simulink model "problem_3"  (R2018a)
settings: Solver=VariableStepAuto  StartTime=0.0  StopTime=10  MaxStep=1e-3  RelTol=1e-3
values from neighbouring files (symbols this model uses):
  a0 = 68 * pi/180    (= 1.18682389136)    [grid_search_minimization.m]    (also in minimization.m = a0Vec(aIdx); problem_1_script.m; problem_3_script.m; smm_params.m)
  dx0 = 1.123    [distance_x.m]    (also in grid_search_minimization.m = sqrt(2/m*(Esys-m*g*y0)); minimization.m = sqrt(2/m*(Esys-m*g*y0)); problem_1_script.m = 5; problem_3_script.m = sqrt(2/m*(Esys-m*g*y0)))
  dy0 = 0    [distance_x.m]    (also in grid_search_minimization.m; minimization.m; problem_1_script.m; problem_3_script.m)
  g = 9.81    [distance_x.m]    (also in grid_search_minimization.m; minimization.m; problem_1_script.m; problem_3_script.m)
  l0 = 0.9937    [distance_x.m]    (also in grid_search_minimization.m = 1; minimization.m = 1; problem_1_script.m = 1; problem_3_script.m = 1)
  m = 80    [distance_x.m]    (also in grid_search_minimization.m; minimization.m; problem_1_script.m; problem_3_script.m)
  x0 = 0    [distance_x.m]    (also in grid_search_minimization.m; minimization.m; problem_1_script.m; problem_3_script.m)
  y0 = l0    (= 0.9937)    [distance_x.m]    (also in grid_search_minimization.m = y0Vec(yIdx); minimization.m = y0Vec(yIdx); problem_1_script.m = 1; problem_3_script.m = y0Vec3(yIdx))
libraries: simulink_extras x1
settings Model: Creator=hgeyer  LastModifiedBy=oliver

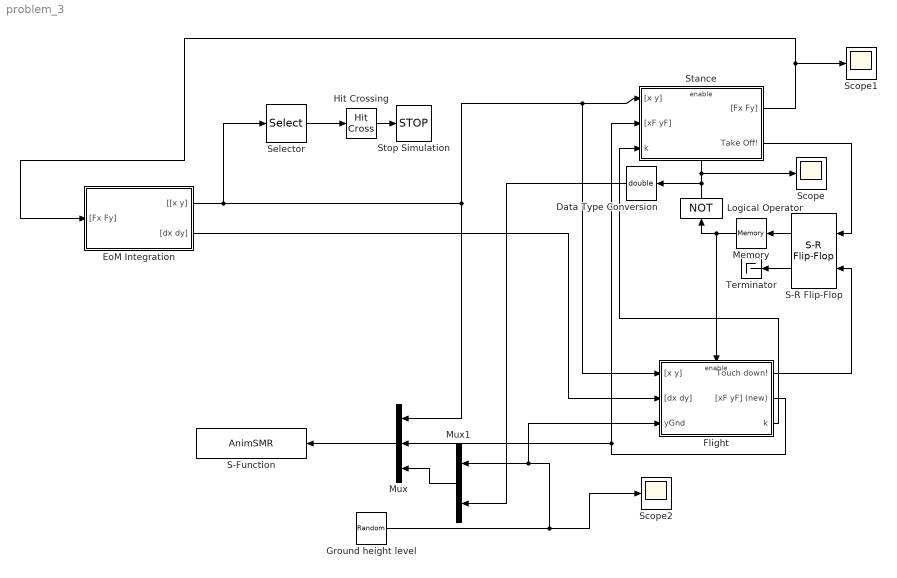
== system problem_3 ==
  " Stance" : Subsystem
  Data Type Conversion : DataTypeConversion  OutDataTypeStr=double
  EoM Integration : Subsystem
  Flight : Subsystem
  Ground height level : UniformRandomNumber  Minimum=-.02  Maximum=.02  SampleTime=0.3
  Hit Crossing : HitCross  HitCrossingDirection=falling
  Logical Operator : Logic  Operator=NOT  AllPortsSameDT=off  OutDataTypeStr=boolean
  Memory : Memory  InitialCondition=1
  Mux : Mux  Inputs=3
  Mux1 : Mux  Inputs=2
  S-Function : S-Function  FunctionName=AnimSMR  Parameters=0.01  SFunctionDeploymentMode=off  EnableBusSupport=off
  S-R Flip-Flop : simulink_extras/Flip Flops/S-R Flip-Flop  initial_condition=1
  Scope : Scope
  Scope1 : Scope
  Scope2 : Scope
  Selector : Selector  InputPortWidth=2  IndexOptions=Index vector (dialog)  Indices=[2]  OutputSizes=1
  Stop Simulation : Stop
  Terminator : Terminator
  wires:
  EoM Integration/1("[[x y]") -> Selector/1, Flight/1("[x y]"), " Stance"/1("[x y]"), Mux/1
  EoM Integration/2("[dx dy]") -> Flight/2("[dx dy]")
  " Stance"/2(Take Off!) -> S-R Flip-Flop/1
  S-R Flip-Flop/1 -> Memory/1
  Logical Operator/1 -> Data Type Conversion/1, " Stance"/Enable, Scope/1
  Memory/1 -> Logical Operator/1, Flight/Enable
  S-R Flip-Flop/2 -> Terminator/1
  Flight/1(Touch down!) -> S-R Flip-Flop/2
  " Stance"/1("[Fx Fy]") -> EoM Integration/1("[Fx Fy]"), Scope1/1
  Flight/2("[xF yF] (new)") -> " Stance"/2("[xF yF]"), Mux/2
  Mux/1 -> S-Function/1
  Mux1/1 -> Mux/3
  Data Type Conversion/1 -> Mux1/2
  Ground height level/1 -> Flight/3(yGnd), Mux1/1, Scope2/1
  Hit Crossing/1 -> Stop Simulation/1
  Selector/1 -> Hit Crossing/1
  Flight/3(k) -> " Stance"/3(k)

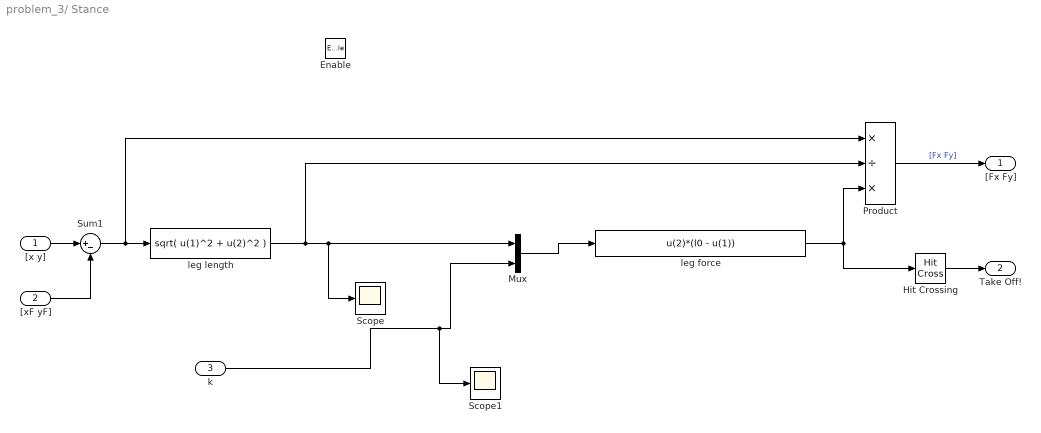
== system problem_3/ Stance ==
  "[x y]" : Inport
  "[xF yF]" : Inport  Port=2
  k : Inport  Port=3
  Enable : EnablePort
  Hit Crossing : HitCross  HitCrossingDirection=falling
  Mux : Mux  Inputs=2
  Product : Product  Inputs=*/*
  Scope : Scope
  Scope1 : Scope
  Sum1 : Sum  Inputs=|+-
  leg force : Fcn  Expr=u(2)*(l0 - u(1))
  leg length : Fcn  Expr=sqrt( u(1)^2 + u(2)^2 )
  "[Fx Fy]" : Outport  OutputWhenDisabled=reset  InitialOutput=[0,0]
  Take Off! : Outport  Port=2  OutputWhenDisabled=reset  InitialOutput=0
  wires:
  Product/1 -> "[Fx Fy]"/1  "[Fx Fy]"
  leg length/1 -> Scope/1, Mux/1, Product/2
  Hit Crossing/1 -> Take Off!/1
  "[x y]"/1 -> Sum1/1
  "[xF yF]"/1 -> Sum1/2
  Sum1/1 -> Product/1, leg length/1
  leg force/1 -> Hit Crossing/1, Product/3
  k/1 -> Scope1/1, Mux/2
  Mux/1 -> leg force/1

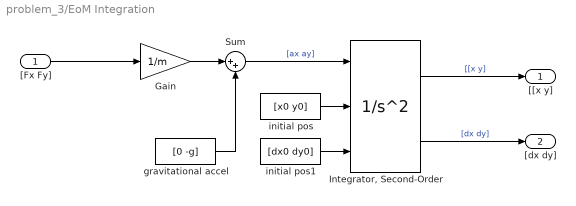
== system problem_3/EoM Integration ==
  "[Fx Fy]" : Inport
  Gain : Gain  Gain=1/m
  "Integrator, Second-Order" : SecondOrderIntegrator  ICSourceX=external  ICSourceDXDT=external
  Sum : Sum  Inputs=|++
  gravitational accel : Constant  Value=[0 -g]
  initial pos : Constant  Value=[x0 y0]
  initial pos1 : Constant  Value=[dx0 dy0]
  "[[x y]" : Outport
  "[dx dy]" : Outport  Port=2
  wires:
  "[Fx Fy]"/1 -> Gain/1
  initial pos1/1 -> "Integrator, Second-Order"/3
  "Integrator, Second-Order"/2 -> "[dx dy]"/1  "[dx dy]"
  Gain/1 -> Sum/1
  initial pos/1 -> "Integrator, Second-Order"/2
  "Integrator, Second-Order"/1 -> "[[x y]"/1  "[[x y]"
  Sum/1 -> "Integrator, Second-Order"/1  "[ax ay]"
  gravitational accel/1 -> Sum/2

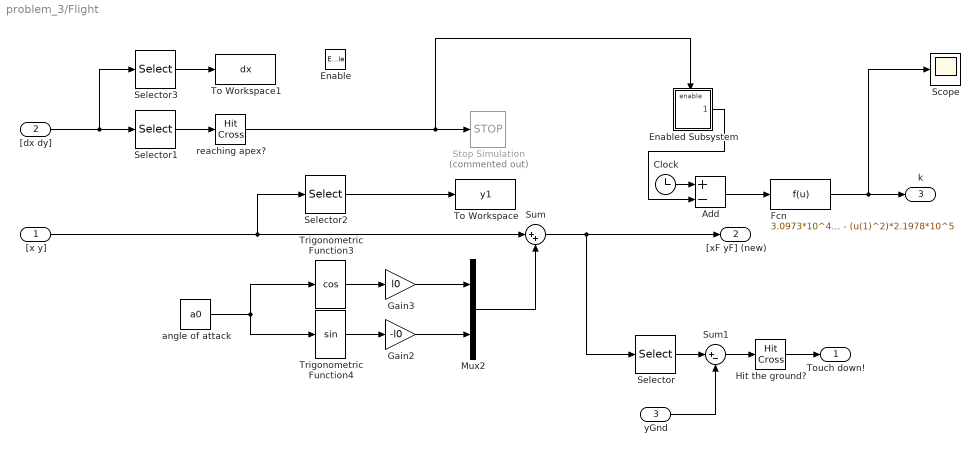
== system problem_3/Flight ==
  "[x y]" : Inport
  "[dx dy]" : Inport  Port=2
  yGnd : Inport  Port=3
  Enable : EnablePort
  Add : Sum  Inputs=+-
  Clock : Clock
  Enabled Subsystem : Subsystem  TreatAsAtomicUnit=on
  Fcn : Fcn  Expr=3.0973*10^4 - (u(1)^2)*2.1978*10^5
  Gain2 : Gain  Gain=-l0
  Gain3 : Gain  Gain=l0
  Hit the ground? : HitCross  HitCrossingDirection=falling
  Mux2 : Mux  Inputs=2
  Scope : Scope
  Selector : Selector  InputPortWidth=2  IndexOptions=Index vector (dialog)  Indices=2  OutputSizes=1
  Selector1 : Selector  InputPortWidth=2  IndexOptions=Index vector (dialog)  Indices=2  OutputSizes=1
  Selector2 : Selector  InputPortWidth=2  IndexOptions=Index vector (dialog)  Indices=2  OutputSizes=1
  Selector3 : Selector  InputPortWidth=2  IndexOptions=Index vector (dialog)  Indices=1  OutputSizes=1
  Stop Simulation : Stop  Commented=on
  Sum : Sum  Inputs=|++
  Sum1 : Sum  Inputs=|+-
  To Workspace : ToWorkspace  VariableName=y1  SampleTime=-1
      settings: MaxDataPoints=1
  To Workspace1 : ToWorkspace  VariableName=dx  SampleTime=-1
  Trigonometric Function3 : Trigonometry  Operator=cos
  Trigonometric Function4 : Trigonometry
  angle of attack : Constant  Value=a0
  reaching apex? : HitCross  HitCrossingOffset=eps  HitCrossingDirection=falling
  Touch down! : Outport  OutputWhenDisabled=reset  InitialOutput=0
  "[xF yF] (new)" : Outport  Port=2
  k : Outport  Port=3
  wires:
  angle of attack/1 -> Trigonometric Function4/1, Trigonometric Function3/1
  Trigonometric Function4/1 -> Gain2/1
  Trigonometric Function3/1 -> Gain3/1
  Gain2/1 -> Mux2/2
  Gain3/1 -> Mux2/1
  Mux2/1 -> Sum/2
  "[x y]"/1 -> Selector2/1, Sum/1
  Sum/1 -> Selector/1, "[xF yF] (new)"/1
  Hit the ground?/1 -> Touch down!/1
  "[dx dy]"/1 -> Selector3/1, Selector1/1
  Selector1/1 -> reaching apex?/1
  reaching apex?/1 -> Enabled Subsystem/Enable, Stop Simulation/1
  Selector2/1 -> To Workspace/1
  Selector3/1 -> To Workspace1/1
  Selector/1 -> Sum1/1
  Sum1/1 -> Hit the ground?/1
  yGnd/1 -> Sum1/2
  Clock/1 -> Add/1
  Add/1 -> Fcn/1
  Enabled Subsystem/1(t_apex) -> Add/2
  Fcn/1 -> Scope/1, k/1

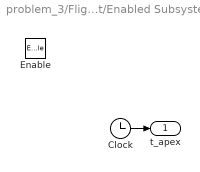
== system problem_3/Flight/Enabled Subsystem ==
  Enable : EnablePort
  Clock : Clock
  t_apex : Outport
  wires:
  Clock/1 -> t_apex/1
